simulink library "LoadProfiles_lib"  (Simulink 8.1)
settings: Solver=ode45  StartTime=0.0  StopTime=10.0  RelTol=1e-3
libraries: rtlab x18
settings Model: Creator=RE25624  LastModifiedBy=pkoralew

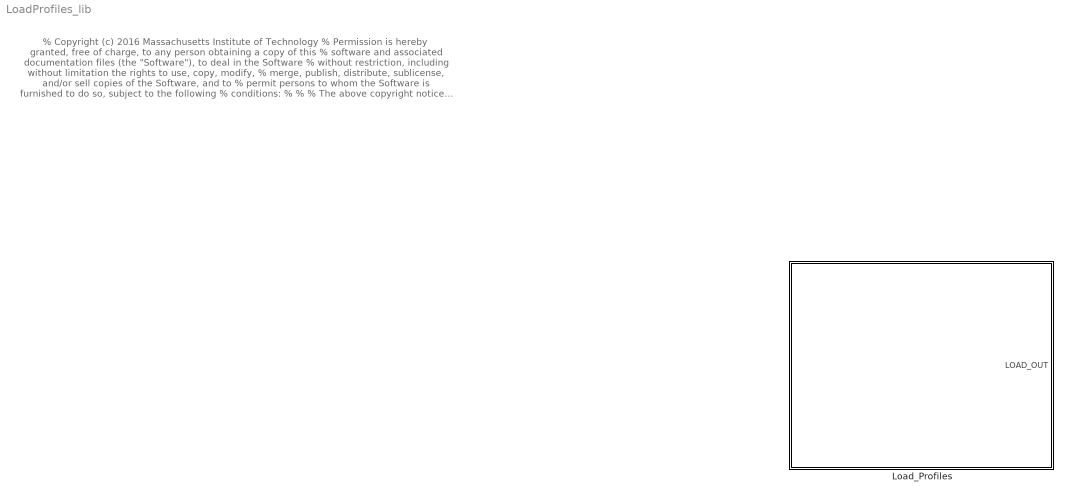
== system LoadProfiles_lib ==
  note: % Copyright (c) 2016 Massachusetts Institute of Technology
      | % Permission is hereby granted, free of charge, to any person obtaining a copy of this
      | % software and associated documentation files (the "Software"), to deal in the Software
      | % without restriction, including without limitation the rights to use, copy, modify,
      | % merge, publish, distribute, sublicense, and/or sell copies of the Software, and to
      | % permit persons to whom the Software is furnished to do so, subject to the following
      | % conditions:
      | %
      | %
      | % The above copyright notice and this permission notice shall be included in
      | % all copies or substantial portions of the Software.
      | %
      | % THE SOFTWARE IS PROVIDED "AS IS", WITHOUT WARRANTY OF ANY KIND, EXPRESS OR IMPLIED,
      | % INCLUDING BUT NOT LIMITED TO THE WARRANTIES OF MERCHANTABILITY, FITNESS FOR A
      | % PARTICULAR PURPOSE AND NONINFRINGEMENT. IN NO EVENT SHALL THE AUTHORS OR COPYRIGHT
      | % HOLDERS BE LIABLE FOR ANY CLAIM, DAMAGES OR OTHER LIABILITY, WHETHER IN AN ACTION
      | % OF CONTRACT, TORT OR OTHERWISE, ARISING FROM, OUT OF OR IN CONNECTION WITH THE
      | % SOFTWARE OR THE USE OR OTHER DEALINGS IN THE SOFTWARE.
      | %
      | %
      | %%
  Load_Profiles : Subsystem

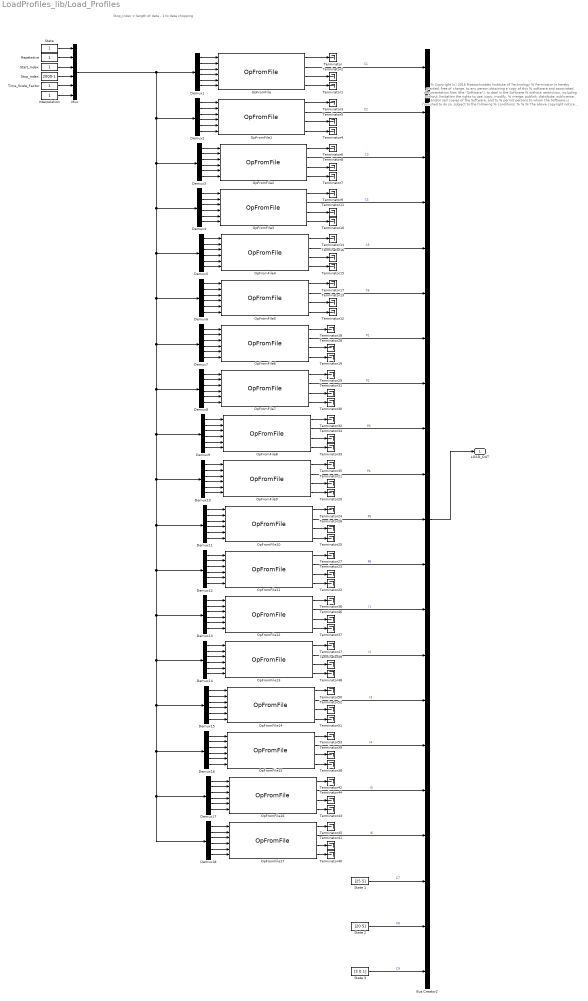
== system LoadProfiles_lib/Load_Profiles ==
  note: Stop_index = length of data - 1 to data chopping
  note: % Copyright (c) 2016 Massachusetts Institute of Technology
      | % Permission is hereby granted, free of charge, to any person obtaining a copy of this
      | % software and associated documentation files (the "Software"), to deal in the Software
      | % without restriction, including without limitation the rights to use, copy, modify,
      | % merge, publish, distribute, sublicense, and/or sell copies of the Software, and to
      | % permit persons to whom the Software is furnished to do so, subject to the following
      | % conditions:
      | %
      | %
      | % The above copyright notice and this permission notice shall be included in
      | % all copies or substantial portions of the Software.
      | %
      | % THE SOFTWARE IS PROVIDED "AS IS", WITHOUT WARRANTY OF ANY KIND, EXPRESS OR IMPLIED,
      | % INCLUDING BUT NOT LIMITED TO THE WARRANTIES OF MERCHANTABILITY, FITNESS FOR A
      | % PARTICULAR PURPOSE AND NONINFRINGEMENT. IN NO EVENT SHALL THE AUTHORS OR COPYRIGHT
      | % HOLDERS BE LIABLE FOR ANY CLAIM, DAMAGES OR OTHER LIABILITY, WHETHER IN AN ACTION
      | % OF CONTRACT, TORT OR OTHERWISE, ARISING FROM, OUT OF OR IN CONNECTION WITH THE
      | % SOFTWARE OR THE USE OR OTHER DEALINGS IN THE SOFTWARE.
      | %
      | %
      | %%
  Bus Creator2 : BusCreator  Inputs=21
  Demux{1..18} (18 alike) : Demux  Outputs=6
  "Interpolation " : Constant
  Mux : Mux  Inputs=6
  OpFromFile : rtlab/DataLogging/OpFromFile  filename_mode=Static (same filename all the time)  reload_mode=Next time model is paused (Real-Time)  init_file_id=0  filename=C1.mat  rtpath='./'  nrtpath='.\'  sample_time=0
  OpFromFile1 : rtlab/DataLogging/OpFromFile  filename_mode=Static (same filename all the time)  reload_mode=Next time model is paused (Real-Time)  init_file_id=0  filename=C2.mat  rtpath='./'  nrtpath='.\'  sample_time=0
  OpFromFile10 : rtlab/DataLogging/OpFromFile  filename_mode=Static (same filename all the time)  reload_mode=Next time model is paused (Real-Time)  init_file_id=0  filename=P5.mat  rtpath='./'  nrtpath='.\'  sample_time=0
  OpFromFile11 : rtlab/DataLogging/OpFromFile  filename_mode=Static (same filename all the time)  reload_mode=Next time model is paused (Real-Time)  init_file_id=0  filename=P6.mat  rtpath='./'  nrtpath='.\'  sample_time=0
  OpFromFile12 : rtlab/DataLogging/OpFromFile  filename_mode=Static (same filename all the time)  reload_mode=Next time model is paused (Real-Time)  init_file_id=0  filename=I1.mat  rtpath='./'  nrtpath='.\'  sample_time=0
  OpFromFile13 : rtlab/DataLogging/OpFromFile  filename_mode=Static (same filename all the time)  reload_mode=Next time model is paused (Real-Time)  init_file_id=0  filename=I2.mat  rtpath='./'  nrtpath='.\'  sample_time=0
  OpFromFile14 : rtlab/DataLogging/OpFromFile  filename_mode=Static (same filename all the time)  reload_mode=Next time model is paused (Real-Time)  init_file_id=0  filename=I3.mat  rtpath='./'  nrtpath='.\'  sample_time=0
  OpFromFile15 : rtlab/DataLogging/OpFromFile  filename_mode=Static (same filename all the time)  reload_mode=Next time model is paused (Real-Time)  init_file_id=0  filename=I4.mat  rtpath='./'  nrtpath='.\'  sample_time=0
  OpFromFile16 : rtlab/DataLogging/OpFromFile  filename_mode=Static (same filename all the time)  reload_mode=Next time model is paused (Real-Time)  init_file_id=0  filename=I5.mat  rtpath='./'  nrtpath='.\'  sample_time=0
  OpFromFile17 : rtlab/DataLogging/OpFromFile  filename_mode=Static (same filename all the time)  reload_mode=Next time model is paused (Real-Time)  init_file_id=0  filename=I6.mat  rtpath='./'  nrtpath='.\'  sample_time=0
  OpFromFile2 : rtlab/DataLogging/OpFromFile  filename_mode=Static (same filename all the time)  reload_mode=Next time model is paused (Real-Time)  init_file_id=0  filename=C3.mat  rtpath='./'  nrtpath='.\'  sample_time=0
  OpFromFile3 : rtlab/DataLogging/OpFromFile  filename_mode=Static (same filename all the time)  reload_mode=Next time model is paused (Real-Time)  init_file_id=0  filename=C4.mat  rtpath='./'  nrtpath='.\'  sample_time=0
  OpFromFile4 : rtlab/DataLogging/OpFromFile  filename_mode=Static (same filename all the time)  reload_mode=Next time model is paused (Real-Time)  init_file_id=0  filename=C5.mat  rtpath='./'  nrtpath='.\'  sample_time=0
  OpFromFile5 : rtlab/DataLogging/OpFromFile  filename_mode=Static (same filename all the time)  reload_mode=Next time model is paused (Real-Time)  init_file_id=0  filename=C6.mat  rtpath='./'  nrtpath='.\'  sample_time=0
  OpFromFile6 : rtlab/DataLogging/OpFromFile  filename_mode=Static (same filename all the time)  reload_mode=Next time model is paused (Real-Time)  init_file_id=0  filename=P1.mat  rtpath='./'  nrtpath='.\'  sample_time=0
  OpFromFile7 : rtlab/DataLogging/OpFromFile  filename_mode=Static (same filename all the time)  reload_mode=Next time model is paused (Real-Time)  init_file_id=0  filename=P2.mat  rtpath='./'  nrtpath='.\'  sample_time=0
  OpFromFile8 : rtlab/DataLogging/OpFromFile  filename_mode=Static (same filename all the time)  reload_mode=Next time model is paused (Real-Time)  init_file_id=0  filename=P3.mat  rtpath='./'  nrtpath='.\'  sample_time=0
  OpFromFile9 : rtlab/DataLogging/OpFromFile  filename_mode=Static (same filename all the time)  reload_mode=Next time model is paused (Real-Time)  init_file_id=0  filename=P4.mat  rtpath='./'  nrtpath='.\'  sample_time=0
  "Repetative " : Constant
  "Start_Index " : Constant
  "State " : Constant
  State 1 : Constant  Value=[25 5]
  State 2 : Constant  Value=[20 5]
  State 3 : Constant  Value=[3 0.1]
  "Stop_Index " : Constant  Value=2000-1
  Terminator{,1..53} (54 alike) : Terminator
  "Time_Scale_Factor " : Constant
  LOAD_OUT : Outport
  wires:
  OpFromFile17/4 -> Terminator40/1
  OpFromFile17/3 -> Terminator41/1
  OpFromFile17/1 -> Terminator45/1
  OpFromFile16/4 -> Terminator43/1
  OpFromFile16/3 -> Terminator44/1
  OpFromFile16/1 -> Terminator42/1
  OpFromFile15/4 -> Terminator38/1
  OpFromFile15/3 -> Terminator39/1
  OpFromFile15/1 -> Terminator53/1
  OpFromFile14/4 -> Terminator51/1
  OpFromFile14/3 -> Terminator52/1
  OpFromFile14/1 -> Terminator50/1
  OpFromFile13/4 -> Terminator48/1
  OpFromFile13/3 -> Terminator49/1
  OpFromFile13/1 -> Terminator47/1
  OpFromFile12/4 -> Terminator37/1
  OpFromFile12/3 -> Terminator46/1
  OpFromFile12/1 -> Terminator36/1
  OpFromFile11/4 -> Terminator22/1
  OpFromFile11/3 -> Terminator23/1
  OpFromFile11/1 -> Terminator27/1
  OpFromFile10/4 -> Terminator25/1
  OpFromFile10/3 -> Terminator26/1
  OpFromFile10/1 -> Terminator24/1
  OpFromFile9/4 -> Terminator20/1
  OpFromFile9/3 -> Terminator21/1
  OpFromFile9/1 -> Terminator35/1
  OpFromFile8/4 -> Terminator33/1
  OpFromFile8/3 -> Terminator34/1
  OpFromFile8/1 -> Terminator32/1
  OpFromFile7/4 -> Terminator30/1
  OpFromFile7/3 -> Terminator31/1
  OpFromFile7/1 -> Terminator29/1
  OpFromFile6/4 -> Terminator19/1
  OpFromFile6/3 -> Terminator28/1
  OpFromFile6/1 -> Terminator18/1
  OpFromFile5/4 -> Terminator12/1
  OpFromFile5/3 -> Terminator13/1
  OpFromFile5/1 -> Terminator17/1
  OpFromFile4/4 -> Terminator15/1
  OpFromFile4/3 -> Terminator16/1
  OpFromFile4/1 -> Terminator14/1
  OpFromFile3/4 -> Terminator10/1
  OpFromFile3/3 -> Terminator11/1
  OpFromFile3/1 -> Terminator9/1
  OpFromFile2/4 -> Terminator7/1
  OpFromFile2/3 -> Terminator8/1
  OpFromFile2/1 -> Terminator6/1
  OpFromFile1/4 -> Terminator4/1
  OpFromFile1/3 -> Terminator5/1
  OpFromFile1/1 -> Terminator3/1
  OpFromFile/4 -> Terminator1/1
  OpFromFile/3 -> Terminator2/1
  OpFromFile/1 -> Terminator/1
  State 3/1 -> Bus Creator2/21  "C9"
  State 2/1 -> Bus Creator2/20  "C8"
  State 1/1 -> Bus Creator2/19  "C7"
  Demux10/3 -> OpFromFile9/3
  Demux10/1 -> OpFromFile9/1
  Demux9/2 -> OpFromFile8/2
  Demux11/1 -> OpFromFile10/1
  Demux9/3 -> OpFromFile8/3
  Demux14/4 -> OpFromFile13/4
  Demux5/4 -> OpFromFile4/4
  Demux9/6 -> OpFromFile8/6
  Demux5/5 -> OpFromFile4/5
  Demux5/3 -> OpFromFile4/3
  Demux11/2 -> OpFromFile10/2
  Demux11/3 -> OpFromFile10/3
  Demux9/1 -> OpFromFile8/1
  Demux14/6 -> OpFromFile13/6
  Demux15/1 -> OpFromFile14/1
  Demux8/6 -> OpFromFile7/6
  Demux10/6 -> OpFromFile9/6
  Demux8/5 -> OpFromFile7/5
  OpFromFile3/2 -> Bus Creator2/4  "C4"
  Demux14/5 -> OpFromFile13/5
  OpFromFile5/2 -> Bus Creator2/6  "C6"
  OpFromFile4/2 -> Bus Creator2/5  "C5"
  "Interpolation "/1 -> Mux/6
  "Stop_Index "/1 -> Mux/4
  "Time_Scale_Factor "/1 -> Mux/5
  OpFromFile2/2 -> Bus Creator2/3  "C3"
  OpFromFile1/2 -> Bus Creator2/2  "C2"
  "Start_Index "/1 -> Mux/3
  OpFromFile/2 -> Bus Creator2/1  "C1"
  "State "/1 -> Mux/1
  "Repetative "/1 -> Mux/2
  Demux3/6 -> OpFromFile2/6
  Demux4/2 -> OpFromFile3/2
  Demux4/1 -> OpFromFile3/1
  Demux9/4 -> OpFromFile8/4
  Demux3/4 -> OpFromFile2/4
  Demux3/3 -> OpFromFile2/3
  Demux3/2 -> OpFromFile2/2
  Demux10/2 -> OpFromFile9/2
  Demux3/5 -> OpFromFile2/5
  Demux1/6 -> OpFromFile/6
  Demux1/5 -> OpFromFile/5
  Demux2/1 -> OpFromFile1/1
  Demux2/2 -> OpFromFile1/2
  Demux10/5 -> OpFromFile9/5
  Demux2/5 -> OpFromFile1/5
  Demux1/4 -> OpFromFile/4
  Demux2/3 -> OpFromFile1/3
  Demux2/4 -> OpFromFile1/4
  Demux3/1 -> OpFromFile2/1
  Demux10/4 -> OpFromFile9/4
  Demux2/6 -> OpFromFile1/6
  Demux1/3 -> OpFromFile/3
  Demux9/5 -> OpFromFile8/5
  Demux4/3 -> OpFromFile3/3
  Demux5/2 -> OpFromFile4/2
  Demux4/5 -> OpFromFile3/5
  Demux4/4 -> OpFromFile3/4
  Demux5/6 -> OpFromFile4/6
  Demux6/1 -> OpFromFile5/1
  Demux6/2 -> OpFromFile5/2
  Demux6/3 -> OpFromFile5/3
  Demux6/4 -> OpFromFile5/4
  Demux8/2 -> OpFromFile7/2
  Demux8/3 -> OpFromFile7/3
  Demux8/4 -> OpFromFile7/4
  Demux7/2 -> OpFromFile6/2
  Demux7/3 -> OpFromFile6/3
  Demux7/4 -> OpFromFile6/4
  Demux6/5 -> OpFromFile5/5
  Demux6/6 -> OpFromFile5/6
  Demux7/1 -> OpFromFile6/1
  Demux8/1 -> OpFromFile7/1
  Demux7/6 -> OpFromFile6/6
  Demux7/5 -> OpFromFile6/5
  Demux1/2 -> OpFromFile/2
  Demux1/1 -> OpFromFile/1
  Demux5/1 -> OpFromFile4/1
  Bus Creator2/1 -> LOAD_OUT/1
  Demux4/6 -> OpFromFile3/6
  Demux11/4 -> OpFromFile10/4
  Demux11/6 -> OpFromFile10/6
  Demux12/1 -> OpFromFile11/1
  Demux13/6 -> OpFromFile12/6
  Demux14/3 -> OpFromFile13/3
  Demux14/1 -> OpFromFile13/1
  Demux12/6 -> OpFromFile11/6
  Demux13/1 -> OpFromFile12/1
  Demux13/3 -> OpFromFile12/3
  Demux13/4 -> OpFromFile12/4
  Demux12/3 -> OpFromFile11/3
  Demux12/4 -> OpFromFile11/4
  Demux14/2 -> OpFromFile13/2
  OpFromFile11/2 -> Bus Creator2/12  "P6"
  Demux16/5 -> OpFromFile15/5
  Demux11/5 -> OpFromFile10/5
  Demux12/5 -> OpFromFile11/5
  Demux12/2 -> OpFromFile11/2
  Demux16/2 -> OpFromFile15/2
  Demux16/3 -> OpFromFile15/3
  Demux16/4 -> OpFromFile15/4
  Demux16/1 -> OpFromFile15/1
  Demux13/5 -> OpFromFile12/5
  Mux/1 -> Demux1/1, Demux2/1, Demux3/1, Demux4/1, Demux7/1, Demux8/1, Demux9/1, Demux10/1, Demux11/1, Demux12/1, Demux13/1, Demux14/1, Demux15/1, Demux16/1, Demux17/1, Demux18/1, Demux6/1, Demux5/1
  Demux15/3 -> OpFromFile14/3
  Demux15/4 -> OpFromFile14/4
  OpFromFile8/2 -> Bus Creator2/9  "P3"
  OpFromFile16/2 -> Bus Creator2/17  "I5"
  OpFromFile7/2 -> Bus Creator2/8  "P2"
  OpFromFile6/2 -> Bus Creator2/7  "P1"
  Demux18/6 -> OpFromFile17/6
  Demux18/5 -> OpFromFile17/5
  Demux18/4 -> OpFromFile17/4
  OpFromFile9/2 -> Bus Creator2/10  "P4"
  OpFromFile10/2 -> Bus Creator2/11  "P5"
  Demux15/5 -> OpFromFile14/5
  Demux15/6 -> OpFromFile14/6
  Demux18/3 -> OpFromFile17/3
  Demux17/5 -> OpFromFile16/5
  Demux18/1 -> OpFromFile17/1
  Demux18/2 -> OpFromFile17/2
  Demux17/6 -> OpFromFile16/6
  Demux17/2 -> OpFromFile16/2
  Demux17/3 -> OpFromFile16/3
  Demux17/1 -> OpFromFile16/1
  Demux17/4 -> OpFromFile16/4
  OpFromFile12/2 -> Bus Creator2/13  "I1"
  Demux15/2 -> OpFromFile14/2
  Demux13/2 -> OpFromFile12/2
  OpFromFile17/2 -> Bus Creator2/18  "I6"
  Demux16/6 -> OpFromFile15/6
  OpFromFile13/2 -> Bus Creator2/14  "I2"
  OpFromFile15/2 -> Bus Creator2/16  "I4"
  OpFromFile14/2 -> Bus Creator2/15  "I3"
